simulink model "Dinamica_numerica_MPC"  (R2024b)
settings: Solver=ode4  StartTime=0.0  StopTime=Durata_sim  FixedStep=step_num  RelTol=1e-6
values from neighbouring files (symbols this model uses):
  a_c0 = 6771    [Propagation_outofplane_transfer.m]
  B_c = C_Dc*S_c/mass_c    (= 0)    [Propagation_outofplane_transfer.m]
  B_d = C_Dd*S_d/mass_d    (= 1.05e-08)    [Propagation_outofplane_transfer.m]
  D = zeros(ny,3)    [final_controller_1deputy2.m]
  delta_a0 = 0    [Propagation_outofplane_transfer.m]
  delta_B = (B_d-B_c)/B_d    (= 1)    [Propagation_outofplane_transfer.m]
  delta_e_x0 = 0    [Propagation_outofplane_transfer.m]
  delta_e_y0 = 0.2/a_c0    (= 2.95377344558e-05)    [Propagation_outofplane_transfer.m]
  delta_i_x0 = 0    [Propagation_outofplane_transfer.m]
  delta_i_y0 = 0.18/a_c0    (= 2.65839610102e-05)    [Propagation_outofplane_transfer.m]
  delta_lambda0 = 0    [Propagation_outofplane_transfer.m]
  e_c0 = 0.001    [Propagation_outofplane_transfer.m]
  i_c0 = 97.05 * pi/180    (= 1.69384203906)    [Propagation_outofplane_transfer.m]
  J_2 = 1.08263e-3    (= 0.00108263)    [Propagation_outofplane_transfer.m]
  M_c0 = 0 * pi/180    (= 0)    [Propagation_outofplane_transfer.m]
  mu = 3.986e5    (= 398600)    [Propagation_outofplane_transfer.m]
  OM_c0 = 30 * pi/180    (= 0.523598775598)    [Propagation_outofplane_transfer.m]
  om_c0 = 90 * pi/180    (= 1.57079632679)    [Propagation_outofplane_transfer.m]
  R_E = 6378    [Propagation_outofplane_transfer.m]
  rho = 1.05259630795205e-3    (= 0.00105259630795)    [Propagation_outofplane_transfer.m]
  ROE_T = [delta_aT,delta_lambdaT,delta_e_xT,delta_e_yT, delta_i_xT, delta_i_yT, delta_B]'    [Propagation_outofplane_transfer.m]
  S_c = 0.1*(1e-3)^2    (= 1e-07)    [Propagation_outofplane_transfer.m]
  S_d = 0.1*(1e-3)^2    (= 1e-07)    [Propagation_outofplane_transfer.m]
  T_orbit = 2*pi/n_c0    [Propagation_outofplane_transfer.m]
  Ts = 100    [Propagation_outofplane_transfer.m]
  u_max = max_thrust/mass_d    (= 3.25e-08)    [Propagation_outofplane_transfer.m]    (also in final_controller_1deputy2.m = 0.0325)
  u_min = min_thrust/mass_d    (= 1.75e-08)    [Propagation_outofplane_transfer.m]    (also in final_controller_1deputy2.m = 0.0175)
undefined symbols (not defined in the file or in its folder): final_controller_1deputy2, inputs4JB2008, JB2008, M_0, OMEGA_c0, omega_c0
libraries: spsMeanLib x6, simulink x3, simulink_extras x2
(part 1 of 4)
settings Model: Creator=giusa  LastModifiedBy=giusa
settings SolverCC: ZeroCrossAlgorithm=Adaptive  EnableFixedStepZeroCrossing=on  MaxZcPerStep=100
settings DebuggingCC: IgnoredZcDiagnostic=none

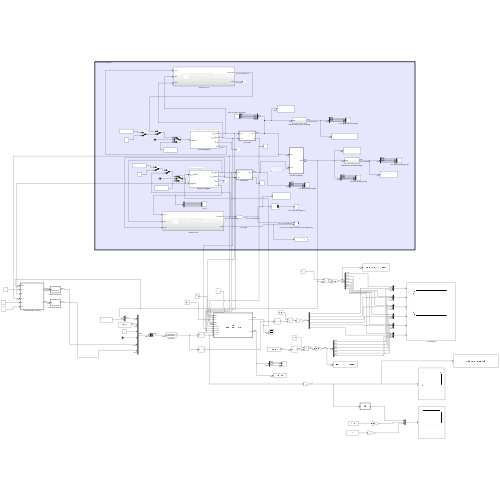
[thumbnail: Simulink's stored preview of the top-level diagram]
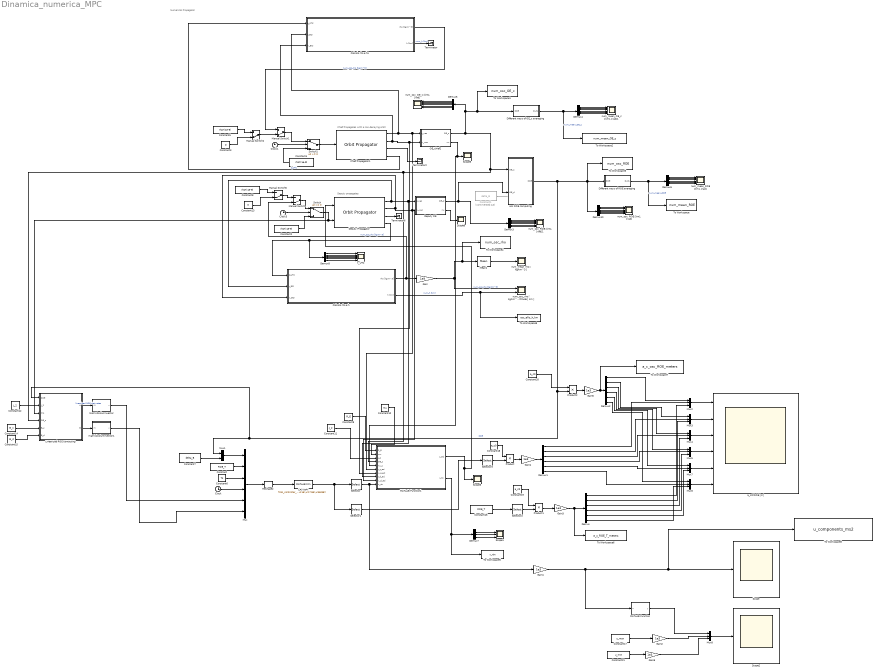
== system Dinamica_numerica_MPC ==
  note: Numerical Propagator
  note: Deputy propagates
  note: Chief Propagates with a non-decaying orbit
  Calcolo rho e h : Subsystem
  Calcolo rho e h1 : Subsystem
  Chief Propagator1 : OrbitPropagator  propagator=Numerical (high precision)  startDate=[2021, 3, 21, 0, 0, 0]  mass=mass_c  action=Error  semiMajorAxis=a_c0  eccentricity=e_c0  inclination=i_c0  raan=OM_c0  argPeriapsis=om_c0  trueAnomaly=nu_c0  inertialPosition=[3649700.0 3308200.0 -4676600.0]  inertialVelocity=[-2750.8 6666.4 2573.4]  fixedPosition=[-4142689.0 -2676864.7 -4669861.6]  fixedVelocity=[1452.7 -6720.7 2568.1]  gravityModel=Oblate ellipsoid (J2)  customR=3396200  customMu=4.305e13  customJ2=1.0826269e-03  customOmega=4.06125949e-3  useEOPs=off  outputTransform=on  useDrag=on  atmosSrc=Port  dragCoeff=C_Dc  dragArea=S_c*(1e3)^2  useEphemerisDateRange=off  includeMoonOccultation=off  reflectivityCoeff=C_R  srpArea=S_c  units=Metric (km/s)  angleUnits=Radians  timeFormat=Gregorian
  Clock : Clock
  Clock1 : Clock
  Clock3 : Clock
  Constant : Constant  Value=ROE_T  VectorParams1D=off
  Constant1 : Constant  Commented=on  Value=delta_B
  Constant10 : Constant  Value=mu
  Constant11 : Constant  Value=J_2
  Constant12 : Constant  Value=J_2
  Constant13 : Constant  Value=0
  Constant14 : Constant  Value=B_c
  Constant15 : Constant  Value=B_d
  Constant16 : Constant  Value=ROE_T  VectorParams1D=off
  Constant17 : Constant  Value=u_max
  Constant18 : Constant  Value=a_c0
  Constant19 : Constant  Value=a_c0
  Constant{2,4..5,8} (4 alike) : Constant  Value=rho*(1e-9)
  Constant20 : Constant  Value=a_c0
  Constant21 : Constant  Value=u_min
  Constant3 : Constant  Value=0
  Constant6 : Constant  Value=Ts
  Constant7 : Constant  Value=delta_B
  Constant9 : Constant  Value=R_E
  Demux{,1..6,8,10} (9 alike) : Demux  Outputs=6
  Demux7 : Demux  Outputs=3
  "Deputy OE " : MATLAB Function  TreatAsAtomicUnit=on
  Deputy Propagator : OrbitPropagator  propagator=Numerical (high precision)  accelIn=on  startDate=[2021, 3, 21, 0, 0, 0]  mass=mass_d  action=Error  semiMajorAxis=a_d0  eccentricity=e_d0  inclination=i_d0  raan=OM_d0  argPeriapsis=om_d0  trueAnomaly=nu_d0  inertialPosition=[3649700.0 3308200.0 -4676600.0]  inertialVelocity=[-2750.8 6666.4 2573.4]  fixedPosition=[-4142689.0 -2676864.7 -4669861.6]  fixedVelocity=[1452.7 -6720.7 2568.1]  gravityModel=Oblate ellipsoid (J2)  customR=3396200  customMu=4.305e13  customJ2=1.0826269e-03  customOmega=4.06125949e-3  useEOPs=off  outputTransform=on  useDrag=on  atmosSrc=Port  dragCoeff=C_Dd  dragArea=S_d*(1e3)^2  useEphemerisDateRange=off  includeMoonOccultation=off  reflectivityCoeff=C_R  srpArea=S_d*(1e3)^2  units=Metric (km/s)  angleUnits=Radians  timeFormat=Gregorian
  Different ways of OE_c averaging : Subsystem
  Different ways of ROE averaging : Subsystem
  Gain : Gain  Gain=1e9
  Gain{1..6} (6 alike) : Gain  Gain=1e3
  LPV MPC : MATLABFcn  MATLABFcn=final_controller_1deputy2(u(1:7),u(8:14),u(15), u(16),u(17:65),u(66:86))  OutputDimensions=10  Output1D=off  SampleTime=Ts
  Linearized ROE computing : MATLAB Function  TreatAsAtomicUnit=on
  MATLAB Function : MATLAB Function  TreatAsAtomicUnit=on
  MATLAB Function1 : MATLAB Function  TreatAsAtomicUnit=on
  Manual Switch{,1..2,5} (4 alike) : ManualSwitch  CurrentSetting=0
  Mean1 : spsMeanLib/Mean  Freq=1/T_orbit  Vinit=rho  Ts=0
  Mux : Mux  Inputs=6
  Mux1 : Mux  Inputs=2
  Mux{2..8} (7 alike) : Mux  Inputs=3
  OE_chief2 : MATLAB Function  TreatAsAtomicUnit=on
  Product : Product
  Product1 : Product
  Product2 : Product
  Reshape2 : Reshape  OutputDimensionality=Column vector (2-D)
  Scope{,2..3,5..6} (5 alike) : Scope
  Scope1 : Scope  NumInputPorts=3
  Selector : Selector  InputPortWidth=10  IndexOptions=Index vector (dialog)  Indices=[1:3]  OutputSizes=1
  Selector1 : Selector  InputPortWidth=10  IndexOptions=Index vector (dialog)  Indices=[4:10]  OutputSizes=1
  Selector2 : Selector  InputPortWidth=7  IndexOptions=Index vector (dialog)  Indices=[1:6]  OutputSizes=1
  Selector3 : Selector  InputPortWidth=7  IndexOptions=Index vector (dialog)  Indices=[1:6]  OutputSizes=1
  Switch : Switch  SaturateOnIntegerOverflow=off  InputSameDT=off
  Switch1 : Switch  SaturateOnIntegerOverflow=off  InputSameDT=off
  Terminator : Terminator
  Terminator2 : Terminator
  Terminator6 : Terminator
  To Workspace : ToWorkspace  VariableName=num_mean_ROE  SaveFormat=Structure With Time  SampleTime=-1
  To Workspace1 : ToWorkspace  VariableName=num_osc_OE_c  SaveFormat=Structure With Time  SampleTime=-1
  To Workspace2 : ToWorkspace  VariableName=num_mean_OE_c  SaveFormat=Structure With Time  SampleTime=-1
  To Workspace3 : ToWorkspace  VariableName=num_osc_ROE  SaveFormat=Structure With Time  SampleTime=-1
  To Workspace4 : ToWorkspace  VariableName=num_osc_rho  SaveFormat=Structure With Time  SampleTime=-1
  To Workspace5 : ToWorkspace  VariableName=r_rtn  SaveFormat=Structure With Time  SampleTime=-1
  To Workspace6 : ToWorkspace  VariableName=a_c_ROE_T_meters  SaveFormat=Structure With Time  SampleTime=-1
  To Workspace7 : ToWorkspace  VariableName=a_c_osc_ROE_meters  SaveFormat=Structure With Time  SampleTime=-1
  To Workspace8 : ToWorkspace  VariableName=u_components_ms2  SaveFormat=Structure With Time  SampleTime=-1
  To Workspace9 : ToWorkspace  VariableName=osc_ellis_h_km  SaveFormat=Structure With Time  SampleTime=-1
  a_c0*ROE [m] : Scope  NumInputPorts=6
  matrix2columnvector : MATLAB Function  TreatAsAtomicUnit=on
  matrix2columnvector1 : MATLAB Function  TreatAsAtomicUnit=on
  "num_mean_OE_c [km], [rad]1" : Scope  NumInputPorts=6
  "num_mean_ROE [km], [rad]" : Scope  NumInputPorts=6
  num_mean_rho [ kg/km^3 ] : Scope
  "num_osc_OE_c [km], [rad]" : Scope  NumInputPorts=6
  "num_osc_ROE [km], [rad]" : Scope  NumInputPorts=6
  "num_osc_ROE [km], [rad]1" : Scope  NumInputPorts=6
  num_osc_rho [ kg/km^3 ] vs num_osc_altitude [ km ] : Scope  NumInputPorts=2
  osc ROE computing : MATLAB Function  TreatAsAtomicUnit=on
  t_UTC : Scope  NumInputPorts=6
  wires:
  Demux6/1 -> "num_mean_ROE [km], [rad]"/1
  Demux6/3 -> "num_mean_ROE [km], [rad]"/3
  Demux6/6 -> "num_mean_ROE [km], [rad]"/6
  Demux6/4 -> "num_mean_ROE [km], [rad]"/4
  Demux6/2 -> "num_mean_ROE [km], [rad]"/2
  Demux6/5 -> "num_mean_ROE [km], [rad]"/5
  Different ways of OE_c averaging/1(Out1) -> To Workspace2/1, Demux4/1  "num_mean_OE_c"
  Demux4/1 -> "num_mean_OE_c [km], [rad]1"/1
  Demux10/4 -> "num_osc_ROE [km], [rad]"/4
  Demux5/2 -> "num_osc_OE_c [km], [rad]"/2
  Demux4/6 -> "num_mean_OE_c [km], [rad]1"/6
  Demux4/2 -> "num_mean_OE_c [km], [rad]1"/2
  Demux8/4 -> t_UTC/4
  Chief Propagator1/3 -> Terminator2/1
  Different ways of ROE averaging/1(Out1) -> To Workspace/1, Demux6/1  "num_mean_ROE"
  Mean1/1 -> num_mean_rho [ kg/km^3 ]/1
  Switch/1 -> Linearized ROE computing/3(rho), Deputy Propagator/2
  Demux5/1 -> "num_osc_OE_c [km], [rad]"/1
  Demux10/6 -> "num_osc_ROE [km], [rad]"/6
  Demux10/5 -> "num_osc_ROE [km], [rad]"/5
  Demux4/4 -> "num_mean_OE_c [km], [rad]1"/4
  Demux4/3 -> "num_mean_OE_c [km], [rad]1"/3
  Demux5/5 -> "num_osc_OE_c [km], [rad]"/5
  Demux10/1 -> "num_osc_ROE [km], [rad]"/1
  Gain/1 -> To Workspace4/1, Mean1/1, num_osc_rho [ kg/km^3 ] vs num_osc_altitude [ km ]/1  "num_osc_rho [kg/km^3]"
  Manual Switch/1 -> Switch/1
  Demux8/3 -> t_UTC/3
  Constant13/1 -> Manual Switch5/2
  Demux8/5 -> t_UTC/5
  Deputy Propagator/4 -> Demux8/1, Calcolo rho e h/1(t_UTC)
  Demux5/4 -> "num_osc_OE_c [km], [rad]"/4
  Clock3/1 -> Switch/2
  Constant2/1 -> Switch/3
  Manual Switch5/1 -> Manual Switch/1
  OE_chief2/2(nu) -> MATLAB Function1/5(nu_c), Scope5/1
  Deputy Propagator/3 -> Terminator6/1
  Demux10/2 -> "num_osc_ROE [km], [rad]"/2
  Calcolo rho e h/1(rho [kg/m^3]) -> Manual Switch/2, Gain/1  "num_osc_rho [kg/m^3]"
  Deputy Propagator/2 -> Calcolo rho e h/3(v_ECI), MATLAB Function1/9(v_d_eci), "Deputy OE "/2(v_vec)
  "Deputy OE "/2(nu) -> Scope6/1
  Demux8/2 -> t_UTC/2
  Chief Propagator1/1 -> MATLAB Function1/6(r_c_eci), OE_chief2/1(r_vec), Calcolo rho e h1/2(r_ECI)
  Demux4/5 -> "num_mean_OE_c [km], [rad]1"/5
  Demux10/3 -> "num_osc_ROE [km], [rad]"/3
  Demux8/1 -> t_UTC/1
  Deputy Propagator/1 -> Calcolo rho e h/2(r_ECI), MATLAB Function1/8(r_d_eci), "Deputy OE "/1(r_vec)
  Calcolo rho e h/2(h [km]) -> To Workspace9/1, num_osc_rho [ kg/km^3 ] vs num_osc_altitude [ km ]/2  "num_h [km]"
  Demux5/6 -> "num_osc_OE_c [km], [rad]"/6
  Demux5/3 -> "num_osc_OE_c [km], [rad]"/3
  OE_chief2/1(OE_c) -> osc ROE computing/1(OE_c), Linearized ROE computing/4(OE_c), MATLAB Function1/4(OE_c), Demux5/1, To Workspace1/1, Different ways of OE_c averaging/1(ROE)
  osc ROE computing/1(ROE) -> Linearized ROE computing/1(ROE), Mux1/1, Product2/2, To Workspace3/1, Demux10/1, Different ways of ROE averaging/1(ROE)  "ROE"
  Constant8/1 -> Manual Switch5/1
  Constant1/1 -> ?
  Chief Propagator1/2 -> MATLAB Function1/7(v_c_eci), OE_chief2/2(v_vec), Calcolo rho e h1/3(v_ECI)
  Demux8/6 -> t_UTC/6
  Demux3/3 -> "num_osc_ROE [km], [rad]1"/3
  "Deputy OE "/1(OE_d) -> Demux3/1, osc ROE computing/2(OE_d)
  Demux3/2 -> "num_osc_ROE [km], [rad]1"/2
  Demux3/6 -> "num_osc_ROE [km], [rad]1"/6
  Demux3/1 -> "num_osc_ROE [km], [rad]1"/1
  Demux3/5 -> "num_osc_ROE [km], [rad]1"/5
  Demux3/4 -> "num_osc_ROE [km], [rad]1"/4
  Constant3/1 -> Manual Switch2/2
  Constant5/1 -> Manual Switch2/1
  Clock1/1 -> Switch1/2
  Manual Switch1/1 -> Switch1/1
  Constant4/1 -> Switch1/3
  Switch1/1 -> Chief Propagator1/1
  Calcolo rho e h1/1(rho [kg/m^3]) -> Manual Switch1/1  "num_osc_rho [kg/m^3]"
  Manual Switch2/1 -> Manual Switch1/2
  Calcolo rho e h1/2(h [km]) -> Terminator/1  "num_h [km]"
  Chief Propagator1/4 -> Calcolo rho e h1/1(t_UTC)  "t_UTC"
  Reshape2/1 -> LPV MPC/1
  Mux/1 -> Reshape2/1
  Linearized ROE computing/2(B) -> matrix2columnvector1/1(M)
  Linearized ROE computing/1(A) -> matrix2columnvector/1(M)  "linearized ROE derivates"
  matrix2columnvector/1(v) -> Mux/5
  matrix2columnvector1/1(v) -> Mux/6
  Constant/1 -> Mux/2
  Clock/1 -> Mux/4
  Constant6/1 -> Mux/3
  Mux1/1 -> Mux/1
  Constant7/1 -> Mux1/2
  MATLAB Function1/1(u_eci) -> Scope3/1, Deputy Propagator/1
  Constant9/1 -> MATLAB Function1/1(R_E)
  Constant10/1 -> MATLAB Function1/2(mu)
  Constant11/1 -> MATLAB Function1/3(J_2)
  Constant12/1 -> Linearized ROE computing/2(J_2)
  Constant14/1 -> Linearized ROE computing/5(B_c)
  Constant15/1 -> Linearized ROE computing/6(B_d)
  Selector/1 -> MATLAB Function1/10(u_rtn), Gain1/1
  Selector1/1 -> Selector3/1
  Mux2/1 -> a_c0*ROE [m]/1
  Mux3/1 -> a_c0*ROE [m]/2
  Mux4/1 -> a_c0*ROE [m]/3
  Mux5/1 -> a_c0*ROE [m]/4
  Mux7/1 -> a_c0*ROE [m]/5
  Mux6/1 -> a_c0*ROE [m]/6
  Demux2/1 -> Mux2/1
  Demux1/1 -> Mux2/2
  Demux/1 -> Mux2/3
  Demux2/2 -> Mux3/1
  Demux1/2 -> Mux3/2
  Demux/2 -> Mux3/3
  Demux2/3 -> Mux4/1
  Demux1/3 -> Mux4/2
  Demux/3 -> Mux4/3
  Demux2/4 -> Mux5/1
  Demux1/4 -> Mux5/2
  Demux/4 -> Mux5/3
  Demux2/5 -> Mux7/1
  Demux1/5 -> Mux7/2
  Demux/5 -> Mux7/3
  Demux2/6 -> Mux6/1
  Demux1/6 -> Mux6/2
  Demux/6 -> Mux6/3
  Gain1/1 -> MATLAB Function/1(u), To Workspace8/1, Scope/1
  Constant17/1 -> Gain2/1
  Mux8/1 -> Scope2/1
  Gain2/1 -> Mux8/2
  MATLAB Function/1(y) -> Mux8/1
  Selector3/1 -> Product/2
  Constant18/1 -> Product/1
  Selector2/1 -> Product1/2
  Product1/1 -> Gain3/1
  Constant19/1 -> Product1/1
  Product2/1 -> Gain5/1
  Constant20/1 -> Product2/1
  Gain3/1 -> To Workspace6/1, Demux/1
  Product/1 -> Gain4/1
  Gain4/1 -> Demux1/1
  Gain5/1 -> To Workspace7/1, Demux2/1
  Constant21/1 -> Gain6/1
  Gain6/1 -> Mux8/3
  LPV MPC/1 -> Selector1/1, Selector/1
  Demux7/1 -> Scope1/1
  Demux7/2 -> Scope1/2
  Demux7/3 -> Scope1/3
  MATLAB Function1/2(r_rtn) -> To Workspace5/1, Demux7/1
  Constant16/1 -> Selector2/1

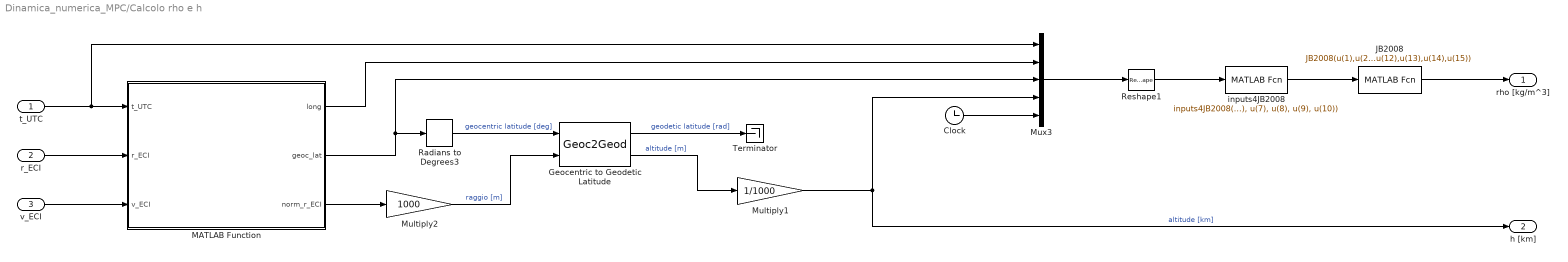
== system Dinamica_numerica_MPC/Calcolo rho e h ==
  t_UTC : Inport
  r_ECI : Inport  Port=2
  v_ECI : Inport  Port=3
  Clock : Clock
  Geocentric to Geodetic Latitude : Geoc2Geod  outputAltitude=on
  JB2008 : MATLABFcn  MATLABFcn=JB2008(u(1),u(2:3),u(4:6),u(7),u(8),u(9),u(10),u(11),u(12),u(13),u(14),u(15))  OutputDimensions=1  Output1D=off
  MATLAB Function : MATLAB Function  TreatAsAtomicUnit=on
  Multiply1 : Gain  Gain=1/1000
  Multiply2 : Gain  Gain=1000
  Mux3 : Mux  Inputs=5
  Radians to Degrees3 : simulink_extras/Transformations/Radians to Degrees
  Reshape1 : Reshape
  Terminator : Terminator
  inputs4JB2008 : MATLABFcn  MATLABFcn=inputs4JB2008(u(1), u(2), u(3), u(4), u(5), u(6), u(7), u(8), u(9), u(10))  OutputDimensions=[1,15]  Output1D=off
  rho [kg/m^3] : Outport
  h [km] : Outport  Port=2
  wires:
  inputs4JB2008/1 -> JB2008/1
  Reshape1/1 -> inputs4JB2008/1
  Mux3/1 -> Reshape1/1
  JB2008/1 -> rho [kg/m^3]/1
  Clock/1 -> Mux3/5
  t_UTC/1 -> MATLAB Function/1(t_UTC), Mux3/1
  v_ECI/1 -> MATLAB Function/3(v_ECI)
  r_ECI/1 -> MATLAB Function/2(r_ECI)
  Multiply1/1 -> h [km]/1, Mux3/4  "altitude [km]"
  Geocentric to Geodetic Latitude/2 -> Multiply1/1  "altitude [m]"
  MATLAB Function/2(geoc_lat) -> Mux3/3, Radians to Degrees3/1
  Multiply2/1 -> Geocentric to Geodetic Latitude/2  "raggio [m]"
  Radians to Degrees3/1 -> Geocentric to Geodetic Latitude/1  "geocentric latitude [deg]"
  Geocentric to Geodetic Latitude/1 -> Terminator/1  "geodetic latitude [rad]"
  MATLAB Function/1(long) -> Mux3/2
  MATLAB Function/3(norm_r_ECI) -> Multiply2/1

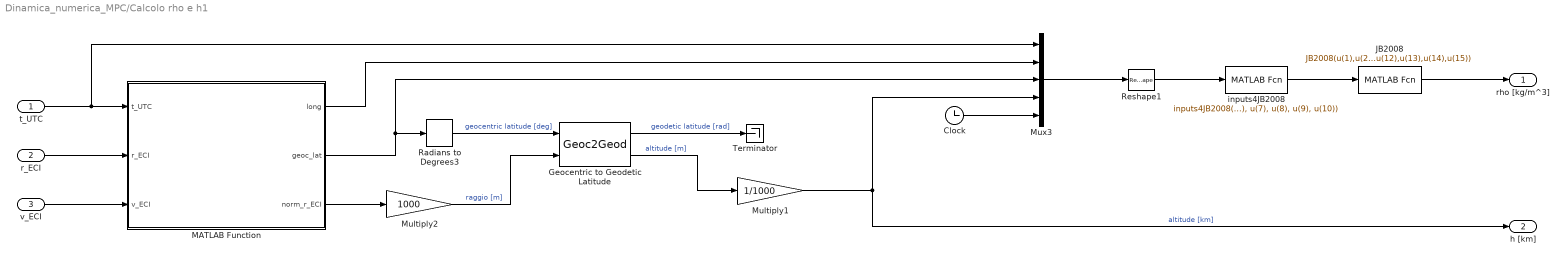
== system Dinamica_numerica_MPC/Calcolo rho e h1 ==
  t_UTC : Inport
  r_ECI : Inport  Port=2
  v_ECI : Inport  Port=3
  Clock : Clock
  Geocentric to Geodetic Latitude : Geoc2Geod  outputAltitude=on
  JB2008 : MATLABFcn  MATLABFcn=JB2008(u(1),u(2:3),u(4:6),u(7),u(8),u(9),u(10),u(11),u(12),u(13),u(14),u(15))  OutputDimensions=1  Output1D=off
  MATLAB Function : MATLAB Function  TreatAsAtomicUnit=on
  Multiply1 : Gain  Gain=1/1000
  Multiply2 : Gain  Gain=1000
  Mux3 : Mux  Inputs=5
  Radians to Degrees3 : simulink_extras/Transformations/Radians to Degrees
  Reshape1 : Reshape
  Terminator : Terminator
  inputs4JB2008 : MATLABFcn  MATLABFcn=inputs4JB2008(u(1), u(2), u(3), u(4), u(5), u(6), u(7), u(8), u(9), u(10))  OutputDimensions=[1,15]  Output1D=off
  rho [kg/m^3] : Outport
  h [km] : Outport  Port=2
  wires:
  MATLAB Function/3(norm_r_ECI) -> Multiply2/1
  MATLAB Function/1(long) -> Mux3/2
  Geocentric to Geodetic Latitude/1 -> Terminator/1  "geodetic latitude [rad]"
  Radians to Degrees3/1 -> Geocentric to Geodetic Latitude/1  "geocentric latitude [deg]"
  Multiply2/1 -> Geocentric to Geodetic Latitude/2  "raggio [m]"
  MATLAB Function/2(geoc_lat) -> Radians to Degrees3/1, Mux3/3
  Geocentric to Geodetic Latitude/2 -> Multiply1/1  "altitude [m]"
  Multiply1/1 -> Mux3/4, h [km]/1  "altitude [km]"
  r_ECI/1 -> MATLAB Function/2(r_ECI)
  v_ECI/1 -> MATLAB Function/3(v_ECI)
  t_UTC/1 -> Mux3/1, MATLAB Function/1(t_UTC)
  Clock/1 -> Mux3/5
  JB2008/1 -> rho [kg/m^3]/1
  Mux3/1 -> Reshape1/1
  Reshape1/1 -> inputs4JB2008/1
  inputs4JB2008/1 -> JB2008/1

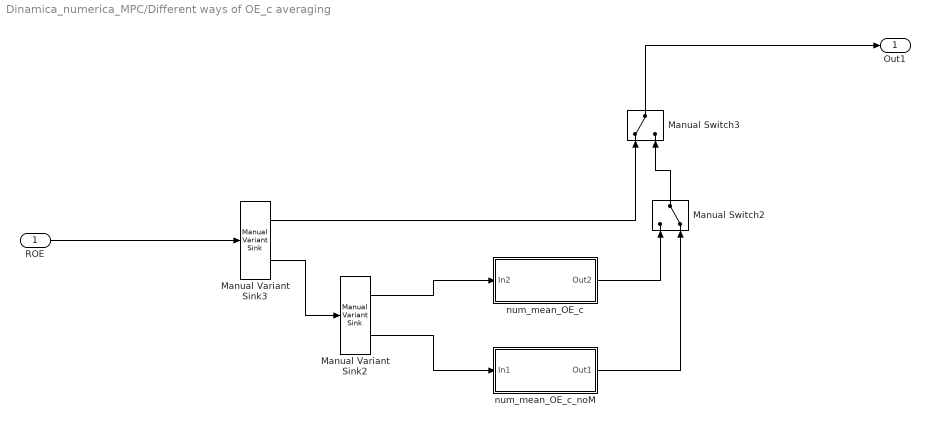
== system Dinamica_numerica_MPC/Different ways of OE_c averaging ==
  ROE : Inport
  Manual Variant Sink2 : simulink/Signal Routing/Manual Variant Sink  NumChoices=2  LabelModeActiveChoice=V_2
  Manual Variant Sink3 : simulink/Signal Routing/Manual Variant Sink  NumChoices=2  LabelModeActiveChoice=V_1
  Manual Switch2 : ManualSwitch  CurrentSetting=0
  Manual Switch3 : ManualSwitch
  num_mean_OE_c : Subsystem
  num_mean_OE_c_noM : Subsystem
  Out1 : Outport
  wires:
  ROE/1 -> Manual Variant Sink3/1
  Manual Variant Sink2/1 -> num_mean_OE_c/1(In2)
  num_mean_OE_c_noM/1(Out1) -> Manual Switch2/2
  Manual Variant Sink3/1 -> Manual Switch3/1
  Manual Switch2/1 -> Manual Switch3/2
  Manual Variant Sink2/2 -> num_mean_OE_c_noM/1(In1)
  Manual Variant Sink3/2 -> Manual Variant Sink2/1
  num_mean_OE_c/1(Out2) -> Manual Switch2/1
  Manual Switch3/1 -> Out1/1

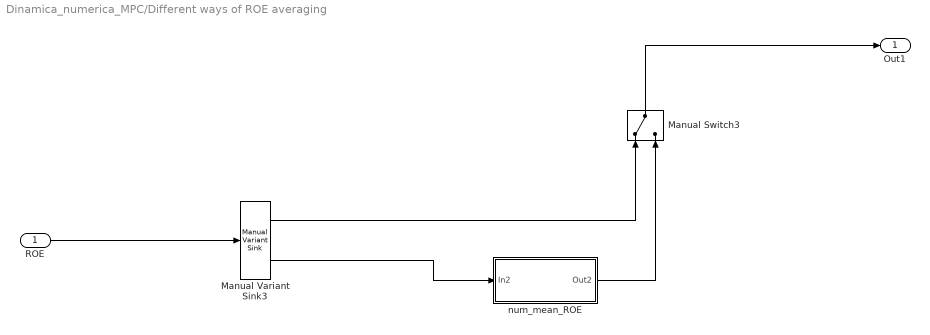
== system Dinamica_numerica_MPC/Different ways of ROE averaging ==
  ROE : Inport
  Manual Variant Sink3 : simulink/Signal Routing/Manual Variant Sink  NumChoices=2  LabelModeActiveChoice=V_1
  Manual Switch3 : ManualSwitch
  num_mean_ROE : Subsystem
  Out1 : Outport
  wires:
  Manual Switch3/1 -> Out1/1
  num_mean_ROE/1(Out2) -> Manual Switch3/2
  Manual Variant Sink3/1 -> Manual Switch3/1
  Manual Variant Sink3/2 -> num_mean_ROE/1(In2)
  ROE/1 -> Manual Variant Sink3/1

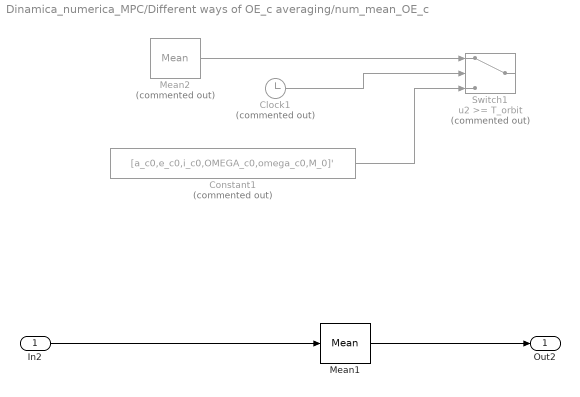
== system Dinamica_numerica_MPC/Different ways of OE_c averaging/num_mean_OE_c ==
  In2 : Inport
  Clock1 : Clock  Commented=on
  Constant1 : Constant  Commented=on  Value=[a_c0,e_c0,i_c0,OMEGA_c0,omega_c0,M_0]'
  Mean1 : spsMeanLib/Mean  Freq=1/(T_orbit)  Vinit=[a_c0,e_c0,i_c0,OM_c0,om_c0,M_c0]'  Ts=0
  Mean2 : spsMeanLib/Mean  Commented=on  Freq=1/T_orbit  Vinit=[a_c0,e_c0,i_c0,OMEGA_c0,omega_c0,M_0]'  Ts=0
  Switch1 : Switch  Commented=on  Threshold=T_orbit  SaturateOnIntegerOverflow=off  InputSameDT=off
  Out2 : Outport
  wires:
  In2/1 -> Mean1/1
  Mean1/1 -> Out2/1
  Constant1/1 -> Switch1/3
  Clock1/1 -> Switch1/2
  Mean2/1 -> Switch1/1

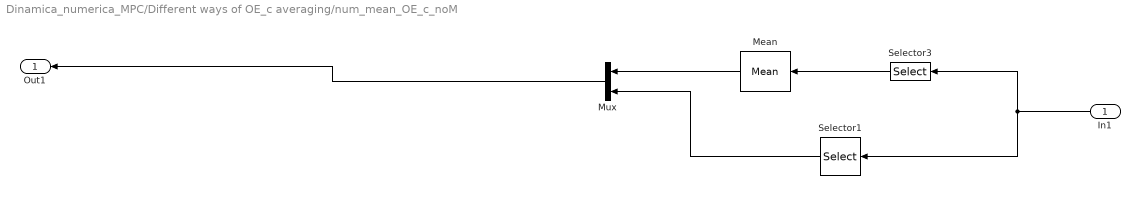
== system Dinamica_numerica_MPC/Different ways of OE_c averaging/num_mean_OE_c_noM ==
  In1 : Inport
  Mean : spsMeanLib/Mean  Freq=1/T_orbit  Vinit=[a_c0,e_c0,i_c0,OM_c0,om_c0]'  Ts=0
  Mux : Mux  Inputs=2
  Selector1 : Selector  InputPortWidth=6  IndexOptions=Index vector (dialog)  Indices=[6]  OutputSizes=1
  Selector3 : Selector  InputPortWidth=6  IndexOptions=Index vector (dialog)  Indices=[1:5]  OutputSizes=1
  Out1 : Outport
  wires:
  In1/1 -> Selector3/1, Selector1/1
  Selector3/1 -> Mean/1
  Selector1/1 -> Mux/2
  Mean/1 -> Mux/1
  Mux/1 -> Out1/1

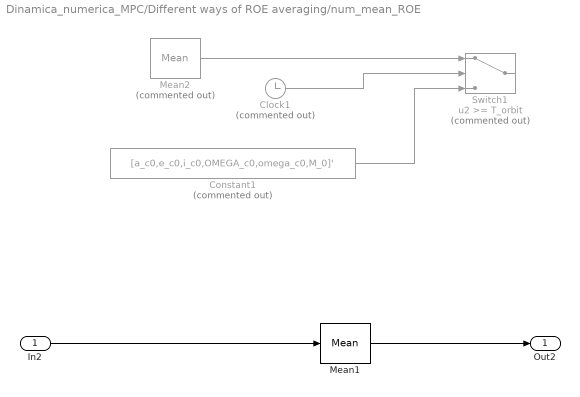
== system Dinamica_numerica_MPC/Different ways of ROE averaging/num_mean_ROE ==
  In2 : Inport
  Clock1 : Clock  Commented=on
  Constant1 : Constant  Commented=on  Value=[a_c0,e_c0,i_c0,OMEGA_c0,omega_c0,M_0]'
  Mean1 : spsMeanLib/Mean  Freq=1/(T_orbit)  Vinit=[delta_a0; delta_lambda0; delta_e_x0; delta_e_y0; delta_i_x0; delta_i_y0]  Ts=0
  Mean2 : spsMeanLib/Mean  Commented=on  Freq=1/T_orbit  Vinit=[a_c0,e_c0,i_c0,OMEGA_c0,omega_c0,M_0]'  Ts=0
  Switch1 : Switch  Commented=on  Threshold=T_orbit  SaturateOnIntegerOverflow=off  InputSameDT=off
  Out2 : Outport
  wires:
  Mean2/1 -> Switch1/1
  Clock1/1 -> Switch1/2
  Constant1/1 -> Switch1/3
  Mean1/1 -> Out2/1
  In2/1 -> Mean1/1

== matlab function Dinamica_numerica_MPC/matrix2columnvector1 ==
  data: M input; v output
function v = fcn(M)
v = rowwise_unroll(M);

== matlab function Dinamica_numerica_MPC/MATLAB Function ==
  data: u input; y output
function y = fcn(u)
y = norm(u);

== matlab function Dinamica_numerica_MPC/Deputy OE  ==
  data: r_vec input; OE_d output; v_vec input; nu output
function [OE_d,nu] = rv2OE(r_vec,v_vec)


oe_type="mean";
mu = 3.986e5; % Gravitational parameter [km^3/s^2]
R_E = 6378; % Mean radius of the Earth [km]

h_vec = cross(r_vec,v_vec); % Angular momentum
h = norm(h_vec,2); % Magnitude of angular momentum
n_vec = cross([0; 0; 1],h_vec); % Mean motion vector
n = norm(n_vec,2); % Magnitude of mean motion vector
v = norm(v_vec,2); % Magnitude of velocity
r = norm(r_vec,2); % Magnitude of position
e_vec = 1/mu.*((v^2 - mu/r).*r_vec - dot(r_vec,v_vec).*v_vec); % Eccentricity vector
e = norm(e_vec,2); % Magnitude of eccentricity

eps = v^2/2 - mu/r; % Specific orbital energy

if (e~=1)
    a = -mu/(2*eps); % Semi-major axis
    p = a*(1-e^2); % Semi-latus rectum
else
    a = Inf; % Parabolic or hyperbolic trajectory
    p = h^2/mu; % Semi-latus rectum for parabolic/hyperbolic trajectory
end

i = acos(h_vec(3)/h); % Inclination
Omega = acos(n_vec(1)/n);
if n_vec(2) < 0
    Omega = 2*pi - Omega; % Adjust for quadrant
end
cos_omega = dot(n_vec,e_vec) / (n * e);
cos_omega = min(1, max(-1, cos_omega));  % Clamping per evitare errori numerici
omega = acos(cos_omega);  % Argument of perigee

if e_vec(3) < 0
    omega = 2*pi - omega; % Adjust for quadrant
end

cos_nu = dot(e_vec,r_vec) / (e * r);
cos_nu = min(1, max(-1, cos_nu));  % Clamping per evitare errori numerici
nu = acos(cos_nu);  % Argument of perigee

if dot(r_vec,v_vec) < 0
    nu = 2*pi - nu; % Adjust for quadrant
end

M = true2mean(nu,e); % Mean anomaly from true anomaly

OE_d = [a, e, i, Omega, omega, M]';


end

== matlab function Dinamica_numerica_MPC/Calcolo rho e h1/MATLAB Function ==
  data: t_UTC input; long output; geoc_lat output; norm_r_ECI output; r_ECI input; v_ECI input
function [long, geoc_lat, norm_r_ECI] = long_lat_h(t_UTC, r_ECI, v_ECI)
year_utc=t_UTC(1);
month_utc=t_UTC(2);
day_utc=t_UTC(3);
hour_utc=t_UTC(4);
min_utc=t_UTC(5);
sec_utc=t_UTC(6);
JD = MVS.date2JD(year_utc, month_utc, day_utc, hour_utc, min_utc, sec_utc);
JD2000=2451545;
alpha_G = JD2alphaG(JD, JD2000, year_utc,month_utc,day_utc,hour_utc,min_utc,sec_utc);
[r_ECEF, v_ECEF] = MVS.ECI2ECEF(r_ECI, v_ECI, alpha_G);
[geoc_lat, long] = ECEF2lat_lon(r_ECEF);
norm_r_ECI = norm(r_ECI,2);

== matlab function Dinamica_numerica_MPC/OE_chief2 ==
  data: r_vec input; OE_c output; v_vec input; nu output
function [OE_c, nu] = rv2OE(r_vec,v_vec)


oe_type="mean";
mu = 3.986e5; % Gravitational parameter [km^3/s^2]
R_E = 6378; % Mean radius of the Earth [km]

h_vec = cross(r_vec,v_vec); % Angular momentum
h = norm(h_vec,2); % Magnitude of angular momentum
n_vec = cross([0; 0; 1],h_vec); % Mean motion vector
n = norm(n_vec,2); % Magnitude of mean motion vector
v = norm(v_vec,2); % Magnitude of velocity
r = norm(r_vec,2); % Magnitude of position
e_vec = 1/mu.*((v^2 - mu/r).*r_vec - dot(r_vec,v_vec).*v_vec); % Eccentricity vector
e = norm(e_vec,2); % Magnitude of eccentricity

eps = v^2/2 - mu/r; % Specific orbital energy

if (e~=1)
    a = -mu/(2*eps); % Semi-major axis
    p = a*(1-e^2); % Semi-latus rectum
else
    a = Inf; % Parabolic or hyperbolic trajectory
    p = h^2/mu; % Semi-latus rectum for parabolic/hyperbolic trajectory
end

i = acos(h_vec(3)/h); % Inclination
Omega = acos(n_vec(1)/n);
if n_vec(2) < 0
    Omega = 2*pi - Omega; % Adjust for quadrant
end
    cos_omega = dot(n_vec,e_vec) / (n * e);
    cos_omega = min(1, max(-1, cos_omega));  % Clamping per evitare errori numerici
    omega = acos(cos_omega);  % Argument of perigee

    if e_vec(3) < 0
        omega = 2*pi - omega; % Adjust for quadrant
    end

cos_nu = dot(e_vec,r_vec) / (e * r);
cos_nu = min(1, max(-1, cos_nu));  % Clamping per evitare errori numerici
nu = acos(cos_nu);  % Argument of perigee

if dot(r_vec,v_vec) < 0
    nu = 2*pi - nu; % Adjust for quadrant
end

M = true2mean(nu,e); % Mean anomaly from true anomaly

OE_c = [a, e, i, Omega, omega, M]';


end

== matlab function Dinamica_numerica_MPC/osc ROE computing ==
  data: OE_c input; ROE output; OE_d input
function ROE = ROE_computing(OE_c, OE_d)

% Chief elements 
a_c=OE_c(1);
e_c=OE_c(2);
i_c=OE_c(3);
OM_c=OE_c(4);
om_c=OE_c(5);
M_c=OE_c(6);

% Deputy elements
a_d=OE_d(1);
e_d=OE_d(2);
i_d=OE_d(3);
OM_d=OE_d(4);
om_d=OE_d(5);
M_d=OE_d(6);

% Mean argument of latitude
u_c=om_c+M_c;
u_d=om_d+M_d;


e_xc=e_c*cos(om_c);
e_yc=e_c*sin(om_c);
e_xd=e_d*cos(om_d);
e_yd=e_d*sin(om_d);

% deltaOE = OE_d-OE_c;

ROE = zeros(6,1);
ROE(1) = (a_d-a_c)/a_c;
ROE(2) = u_d-u_c+(OM_d-OM_c)*cos(i_c);
ROE(3) = e_xd - e_xc;
ROE(4) = e_yd - e_yc;
ROE(5) = i_d - i_c;
ROE(6) = (OM_d - OM_c)*sin(i_c);
% ROE(7) = delta_B;

end
